simulink model "power_twelvepulses"  (Simulink 6.0)
settings: Solver=ode23tb  StartTime=0.0  StopTime=.05  RelTol=1e-3
undefined symbols (not defined in the file or in its folder): D1, Delta
libraries: powerlib x17, powerlib_extras x1
settings Model: Creator=dkennedy  LastModifiedBy=batserve  ExtModeAutoUpdateStatusClock=off
settings DataIOCC: SignalLoggingName=sigsOut
settings OptimizationCC: BlockReduction=off  BooleanDataType=off
settings DebuggingCC: SolverPrmCheckMsg=none
settings HardwareCC: TargetUnknown=on

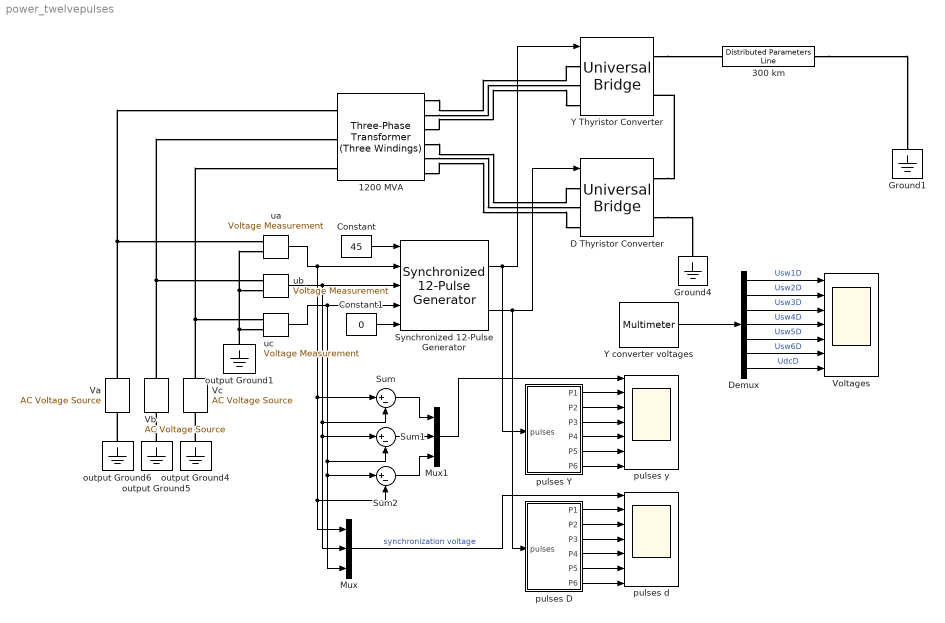
== system power_twelvepulses ==
  " Synchronized 12-Pulse Generator" : powerlib_extras/Control  Blocks/ Synchronized 12-Pulse Generator  freq=60  pwidth=20  Double_Pulse=off
  1200 MVA : powerlib/Elements/Three-Phase Transformer (Three Windings)  NominalPower=[ 1200e6 , 60 ]  Winding1Connection=Yg  Winding1="[ 500e3 0  0 ]"  Winding2Connection=Y  Winding2=[ 200e3 0 0]  Winding3Connection=Delta (D1)  Winding3=[ 200e3 0.001 0]  SetSaturation=off  Rm=500  Lm=500  Saturation=[0 0; 1 1.2; 2 1.1]  Hysteresis=off  DataFile='basic_model'  SetInitialFlux=off  InitialFluxes=[0.8 -0.8 0.7]  Measurements=None  TransfoNumber=0
      settings: AttributesFormatString=\n
  300 km : powerlib/Elements/Distributed Parameters Line  Phases=1  Frequency=60  Resistance=0.015  Inductance=0.792e-3  Capacitance=14.4e-9  Length=300  x1=[0 0 0 0; 0.0001244 0 0 0; 0.0002488 0 0 0; 0.0003733 0 0 0; 0.0004977 0 0 0; 0.0006221 0 0 0]  x2=[0 0 0 0; 0.0001244 0 0 0; 0.0002488 0 0 0; 0.0003733 0 0 0; 0.0004977 0 0 0; 0.0006221 0 0 0]  x3=[0 0 0 0; 0.0001244 0 0 0; 0.0002488 0 0 0; 0.0003733 0 0 0; 0.0004977 0 0 0; 0.0006221 0 0 0]  x4=[0 0 0 0; 0.0001244 0 0 0; 0.0002488 0 0 0; 0.0003733 0 0 0; 0.0004977 0 0 0; 0.0006221 0 0 0]  x5=0  Measurements=Phase-to-ground voltages
      settings: AttributesFormatString=\n
  Constant : Constant  Value=45
  Constant1 : Constant  Value=0
  D Thyristor Converter : powerlib/Power Electronics/Universal Bridge  Arms=3  SnubberResistance=2000  SnubberCapacitance=inf  Device=Thyristors  Ron=1e-3  Lon=0  ForwardVoltages="[  0.8  0.8  ]"  ForwardVoltage=0  GTOparameters=[ 10e-6 , 20e-6 ]  IGBTparameters=[ 1e-6 , 2e-6 ]  Measurements=All voltages and currents
  Demux : Demux  Outputs=7
  Ground1 : powerlib/Elements/Ground  Orientation=down  PhysicalDomain=powersysdomain  SubClassName=unknown  LeftPortType=p1  RightPortType=p1  LConnTagsString=a
  Ground4 : powerlib/Elements/Ground  Orientation=down  PhysicalDomain=powersysdomain  SubClassName=unknown  LeftPortType=p1  RightPortType=p1  LConnTagsString=a
  Mux : Mux  Inputs=3
  Mux1 : Mux  Inputs=3
  Sum : Sum  Inputs=|+-  SaturateOnIntegerOverflow=on  InputSameDT=on
  Sum1 : Sum  Inputs=|+-  SaturateOnIntegerOverflow=on  InputSameDT=on
  Sum2 : Sum  Inputs=|+-  SaturateOnIntegerOverflow=on  InputSameDT=on
  Va : powerlib/Electrical Sources/AC Voltage Source  Description=source block  Orientation=up  Amplitude=500e3/sqrt(3)*sqrt(2)  Phase=0  Frequency=60  SampleTime=0  Measurements=None
      settings: AttributesFormatString=\n
  Vb : powerlib/Electrical Sources/AC Voltage Source  Description=source block  Orientation=up  Amplitude=500e3/sqrt(3)*sqrt(2)  Phase=-120  Frequency=60  SampleTime=0  Measurements=None
      settings: AttributesFormatString=\n
  Vc : powerlib/Electrical Sources/AC Voltage Source  Description=source block  Orientation=up  Amplitude=500e3/sqrt(3)*sqrt(2)  Phase=120  Frequency=60  SampleTime=0  Measurements=None
      settings: AttributesFormatString=\n
  Voltages : Scope  NumInputPorts=7
      settings: TimeRange=0.035  YMin=-400~-1~-1~-1~0~0~0  YMax=400~1~1~1~1~1~1  SaveName=VI_scope2  SampleInput=on  SampleTime=1/60/512
  Y Thyristor Converter : powerlib/Power Electronics/Universal Bridge  Arms=3  SnubberResistance=2000  SnubberCapacitance=.1e-6  Device=Thyristors  Ron=1e-3  Lon=0  ForwardVoltages="[  0.8  0.8  ]"  ForwardVoltage=0  GTOparameters=[ 10e-6 , 20e-6 ]  IGBTparameters=[ 1e-6 , 2e-6 ]  Measurements=All voltages and currents
  "Y converter voltages " : powerlib/Measurements/Multimeter  Tag=PoWeRsYsTeMmEaSuReMeNt  PhasorSimulation=off  OutputType=Magnitude  sel=[1 2 3 4 5 6 21]  L=34  Gain=[-1 -1 -1 -1 -1 -1 1]  yselected={'Usw1: D Thyristor Converter','Usw2: D Thyristor Converter','Usw3: D Thyristor Converter','Usw4: D Thyristor Converter','Usw5: D Thyristor Converter','Usw6: D Thyristor Converter','Us_ph1_gnd: 300 km'};  PSBOutputType=1  PSBequivalent=0  AxesSetting=[0,0.1,-100,100]  Display=0  SavedBlockNames=-11
      settings: AttributesFormatString=\n
  output Ground{1,4..6} (4 alike) : powerlib/Elements/Ground  Orientation=down  PhysicalDomain=powersysdomain  SubClassName=unknown  LeftPortType=p1  RightPortType=p1  LConnTagsString=a
  pulses D : Subsystem
  pulses Y : Subsystem
  pulses d : Scope  NumInputPorts=7
      settings: TimeRange=0.035  YMin=-500000~0~0~0~0~0~0  YMax=500000~1~1~1~1~1~1  SaveName=VI_scope1  SampleInput=on  SampleTime=1/60/512
  pulses y : Scope  NumInputPorts=7
      settings: TimeRange=0.1  YMin=-500000~0~0~0~0~0~0  YMax=500000~1~1~1~1~1~1  SaveName=VI_scope  SampleInput=on  SampleTime=1/60/512
  ua : powerlib/Measurements/Voltage Measurement  Tag=PoWeRsYsTeMmEaSuReMeNt  PhasorSimulation=off  OutputType=Magnitude  PSBequivalent=0
  ub : powerlib/Measurements/Voltage Measurement  Tag=PoWeRsYsTeMmEaSuReMeNt  PhasorSimulation=off  OutputType=Magnitude  PSBequivalent=0
  uc : powerlib/Measurements/Voltage Measurement  Tag=PoWeRsYsTeMmEaSuReMeNt  PhasorSimulation=off  OutputType=Magnitude  PSBequivalent=0
  wires:
  Constant1/1 -> " Synchronized 12-Pulse Generator"/5
  pulses D/6(P6) -> pulses d/7
  pulses D/1(P1) -> pulses d/2
  pulses D/2(P2) -> pulses d/3
  pulses D/3(P3) -> pulses d/4
  pulses D/4(P4) -> pulses d/5
  pulses D/5(P5) -> pulses d/6
  Mux/1 -> pulses d/1  "synchronization voltage"
  Sum/1 -> Mux1/1
  Sum1/1 -> Mux1/2
  Sum2/1 -> Mux1/3
  Mux1/1 -> pulses y/1
  Constant/1 -> " Synchronized 12-Pulse Generator"/1
  pulses Y/1(P1) -> pulses y/2
  pulses Y/2(P2) -> pulses y/3
  pulses Y/3(P3) -> pulses y/4
  pulses Y/4(P4) -> pulses y/5
  pulses Y/5(P5) -> pulses y/6
  pulses Y/6(P6) -> pulses y/7
  ua/1 -> " Synchronized 12-Pulse Generator"/2, Sum/1, Mux/1, Sum2/2
  ub/1 -> " Synchronized 12-Pulse Generator"/3, Sum/2, Mux/2, Sum1/1
  uc/1 -> " Synchronized 12-Pulse Generator"/4, Sum1/2, Mux/3, Sum2/1
  " Synchronized 12-Pulse Generator"/1 -> Y Thyristor Converter/1, pulses Y/1(pulses)
  " Synchronized 12-Pulse Generator"/2 -> pulses D/1(pulses), D Thyristor Converter/1
  Demux/1 -> Voltages/1  "Usw1D"
  Demux/2 -> Voltages/2  "Usw2D"
  Demux/3 -> Voltages/3  "Usw3D"
  Demux/4 -> Voltages/4  "Usw4D"
  Demux/5 -> Voltages/5  "Usw5D"
  Demux/6 -> Voltages/6  "Usw6D"
  Demux/7 -> Voltages/7  "UdcD"
  "Y converter voltages "/1 -> Demux/1
  connections:
  output Ground6/LConn1 -- Va/LConn1
  output Ground5/LConn1 -- Vb/LConn1
  output Ground4/LConn1 -- Vc/LConn1
  Vc/RConn1 -- uc/LConn1 -- 1200 MVA/LConn3
  Vb/RConn1 -- ub/LConn1 -- 1200 MVA/LConn2
  Va/RConn1 -- ua/LConn1 -- 1200 MVA/LConn1
  output Ground1/LConn1 -- ua/LConn2 -- ub/LConn2 -- uc/LConn2
  D Thyristor Converter/RConn1 -- Y Thyristor Converter/RConn2
  D Thyristor Converter/RConn2 -- Ground4/LConn1
  1200 MVA/RConn2 -- Y Thyristor Converter/LConn2
  1200 MVA/RConn1 -- Y Thyristor Converter/LConn1
  1200 MVA/RConn3 -- Y Thyristor Converter/LConn3
  Y Thyristor Converter/RConn1 -- 300 km/LConn1
  300 km/RConn1 -- Ground1/LConn1
  1200 MVA/RConn4 -- D Thyristor Converter/LConn1
  1200 MVA/RConn5 -- D Thyristor Converter/LConn2
  1200 MVA/RConn6 -- D Thyristor Converter/LConn3

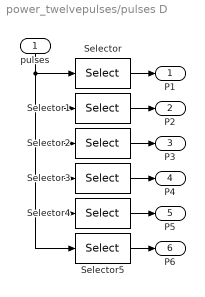
== system power_twelvepulses/pulses D ==
  pulses : Inport  Orientation=down  Port=1  LatchInput=off
  Selector : Selector  InputPortWidth=6
  Selector1 : Selector  Elements=2  InputPortWidth=6
  Selector2 : Selector  Elements=3  InputPortWidth=6
  Selector3 : Selector  Elements=4  InputPortWidth=6
  Selector4 : Selector  Elements=5  InputPortWidth=6
  Selector5 : Selector  Elements=6  InputPortWidth=6
  P1 : Outport
  P2 : Outport  Port=2
  P3 : Outport  Port=3
  P4 : Outport  Port=4
  P5 : Outport  Port=5
  P6 : Outport  Port=6
  wires:
  Selector/1 -> P1/1
  pulses/1 -> Selector4/1, Selector5/1, Selector3/1, Selector2/1, Selector1/1, Selector/1
  Selector1/1 -> P2/1
  Selector2/1 -> P3/1
  Selector3/1 -> P4/1
  Selector4/1 -> P5/1
  Selector5/1 -> P6/1

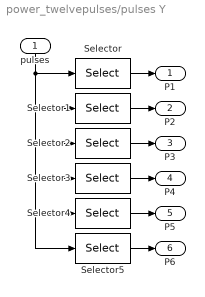
== system power_twelvepulses/pulses Y ==
  pulses : Inport  Orientation=down  Port=1  LatchInput=off
  Selector : Selector  InputPortWidth=6
  Selector1 : Selector  Elements=2  InputPortWidth=6
  Selector2 : Selector  Elements=3  InputPortWidth=6
  Selector3 : Selector  Elements=4  InputPortWidth=6
  Selector4 : Selector  Elements=5  InputPortWidth=6
  Selector5 : Selector  Elements=6  InputPortWidth=6
  P1 : Outport
  P2 : Outport  Port=2
  P3 : Outport  Port=3
  P4 : Outport  Port=4
  P5 : Outport  Port=5
  P6 : Outport  Port=6
  wires:
  Selector5/1 -> P6/1
  Selector4/1 -> P5/1
  Selector3/1 -> P4/1
  Selector2/1 -> P3/1
  Selector1/1 -> P2/1
  pulses/1 -> Selector/1, Selector1/1, Selector2/1, Selector3/1, Selector5/1, Selector4/1
  Selector/1 -> P1/1
